simulink model "Gimbal"  (R2025b)
settings: Solver=FixedStepAuto  StartTime=0.0  StopTime=10.0  RelTol=1e-3
undefined symbols (not defined in the file): s_gimbal_angles
settings Model: DataDictionary=Gimbal_data.sldd  Creator=mauro  LastModifiedBy=mauro

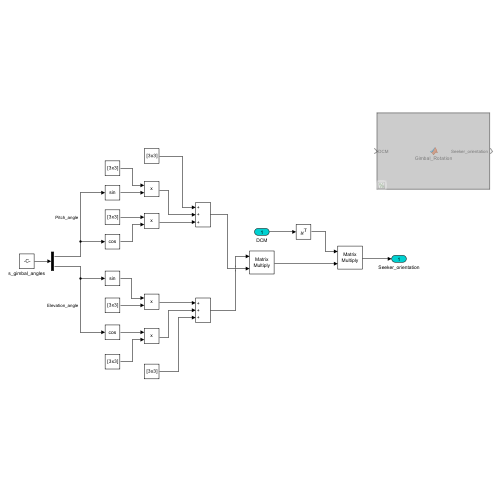
[thumbnail: Simulink's stored preview of the top-level diagram]
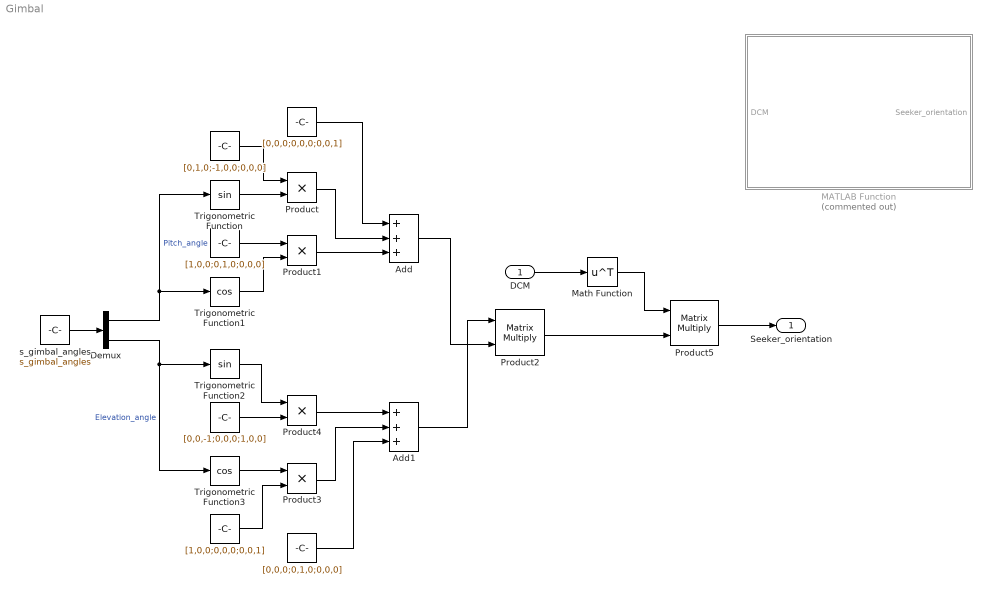
== system Gimbal ==
  DCM : Inport  PortDimensions=[3 3]
  " " : Constant  Value=[0,1,0;-1,0,0;0,0,0]
  "  " : Constant  Value=[1,0,0;0,1,0;0,0,0]
  "   " : Constant  Value=[0,0,0;0,0,0;0,0,1]
  "     " : Constant  Value=[0,0,0;0,1,0;0,0,0]
  "      " : Constant  Value=[1,0,0;0,0,0;0,0,1]
  "       " : Constant  Value=[0,0,-1;0,0,0;1,0,0]
  Add : Sum  Inputs=+++
  Add1 : Sum  Inputs=+++
  Demux : Demux  Outputs=2
  MATLAB Function : MATLAB Function  Commented=on  TreatAsAtomicUnit=on
  Math Function : Math  Operator=transpose
  Product{,1,3..4} (4 alike) : Product
  Product2 : Product  Multiplication=Matrix(*)
  Product5 : Product  Multiplication=Matrix(*)
  Trigonometric Function : Trigonometry
  Trigonometric Function1 : Trigonometry  Operator=cos
  Trigonometric Function2 : Trigonometry
  Trigonometric Function3 : Trigonometry  Operator=cos
  s_gimbal_angles : Constant  Value=s_gimbal_angles
  Seeker_orientation : Outport
  wires:
  s_gimbal_angles/1 -> Demux/1
  Demux/1 -> Trigonometric Function/1, Trigonometric Function1/1  "Pitch_angle"
  Demux/2 -> Trigonometric Function3/1, Trigonometric Function2/1  "Elevation_angle"
  " "/1 -> Product/1
  Trigonometric Function/1 -> Product/2
  "  "/1 -> Product1/1
  Trigonometric Function1/1 -> Product1/2
  Product/1 -> Add/2
  "   "/1 -> Add/1
  Product1/1 -> Add/3
  "      "/1 -> Product3/2
  Trigonometric Function3/1 -> Product3/1
  Trigonometric Function2/1 -> Product4/1
  "       "/1 -> Product4/2
  Product3/1 -> Add1/2
  Product4/1 -> Add1/1
  "     "/1 -> Add1/3
  Product2/1 -> Product5/2
  Add1/1 -> Product2/1
  Add/1 -> Product2/2
  DCM/1 -> Math Function/1
  Math Function/1 -> Product5/1
  Product5/1 -> Seeker_orientation/1

== matlab function Gimbal/MATLAB Function ==
  data: Seeker_orientation output; DCM input; s_gimbal_angles parameter
function Seeker_orientation = Gimbal_Rotation(DCM, s_gimbal_angles)

Pitch_angle     = s_gimbal_angles(1);
Elevation_angle = s_gimbal_angles(2);

Seeker_local = [cos(Elevation_angle),0,-sin(Elevation_angle);...
                      0,1,0;...
                      sin(Elevation_angle),0,cos(Elevation_angle)]*[cos(Pitch_angle),sin(Pitch_angle),0;...
                                                     -sin(Pitch_angle),cos(Pitch_angle),0;...
                                                     0,0,1];

Seeker_orientation = DCM'*Seeker_local;
